simulink model "Pedal_Interpretation_exe"  (Simulink 7.0)
settings: Solver=ode4  StartTime=0.0  StopTime=88  FixedStep=0.01  RelTol=1e-3
InitFcn:
  | PedalInterp_para
values from neighbouring files (symbols this model uses):
  ped_min = 5    [PedalInterp_para.m]
  T_max_Brake = 4000    [PedalInterp_para.m]
  TI = 0    [PAS_callback.m]
undefined symbols (not defined in the file or in its folder): fzgbib, m_ab_100pro, m_ab_70pro, PedalInterpretation, v_bereich
libraries: simulink x320
(part 4 of 23)

== system Pedal_Interpretation_exe/TestData 1/SR-PI-02.2 Acceleration pedal interpretation/v = const & phi_Acc = const/Generate constant 6 ==
  Generate  constant for partition1 variant1 1 : Subsystem  mask(Feature generation){X0=0, T=2}
      mask prompts: X0 "Constant value:"; T "Duration"
      mask help: Output a decreasing ramp signal limited from bottom and top, starting at the specified time.
      mask Display: plot([1:2],[4,4])
  Generate  constant for partition1 variant2 1 : Subsystem  mask(Feature generation){X0=100, T=2}
      mask prompts: X0 "Constant value:"; T "Duration"
      mask help: Output a decreasing ramp signal limited from bottom and top, starting at the specified time.
      mask Display: plot([1:2],[4,4])
  Generate  constant for partition1 variant3 1 : Subsystem  mask(Feature generation){X0=50, T=2}
      mask prompts: X0 "Constant value:"; T "Duration"
      mask help: Output a decreasing ramp signal limited from bottom and top, starting at the specified time.
      mask Display: plot([1:2],[4,4])
  TestDataVariants Sequence : Subsystem
  switch : MultiPortSwitch  Inputs=3  OutDataType=sfix(16)  OutScaling=2^0
  phi_Acc : Outport  OutDataType=sfix(16)  OutScaling=2^0
  wires:
  switch/1 -> phi_Acc/1
  Generate  constant for partition1 variant2 1/1(Out1) -> switch/3
  Generate  constant for partition1 variant1 1/1(Out1) -> switch/2
  Generate  constant for partition1 variant3 1/1(Out1) -> switch/4
  TestDataVariants Sequence/1(Out1) -> switch/1

== system Pedal_Interpretation_exe/TestData 1/SR-PI-02.2 Acceleration pedal interpretation/v = const & phi_Acc decreases & T_des_Drive < 0/Bound Precond2 ==
  Signal : Inport  OutDataType=sfix(16)  OutScaling=2^0
  Reference : Inport  Port=2  OutDataType=sfix(16)  OutScaling=2^0
  RelOp : RelationalOperator  Operator=<  LogicOutDataTypeMode=Specify via dialog
  Activate : Outport  OutDataType=sfix(16)  OutScaling=2^0
  wires:
  Signal/1 -> RelOp/1
  RelOp/1 -> Activate/1
  Reference/1 -> RelOp/2

== system Pedal_Interpretation_exe/TestData 1/SR-PI-02.2 Acceleration pedal interpretation/v = const & phi_Acc decreases & T_des_Drive < 0/Generate constant 6 ==
  Generate  constant for partition1 variant1 1 : Subsystem  mask(Feature generation){X0=-10, T=2}
      mask prompts: X0 "Constant value:"; T "Duration"
      mask help: Output a decreasing ramp signal limited from bottom and top, starting at the specified time.
      mask Display: plot([1:2],[4,4])
  Generate  constant for partition1 variant2 1 : Subsystem  mask(Feature generation){X0=70, T=2}
      mask prompts: X0 "Constant value:"; T "Duration"
      mask help: Output a decreasing ramp signal limited from bottom and top, starting at the specified time.
      mask Display: plot([1:2],[4,4])
  Generate  constant for partition1 variant3 1 : Subsystem  mask(Feature generation){X0=0, T=2}
      mask prompts: X0 "Constant value:"; T "Duration"
      mask help: Output a decreasing ramp signal limited from bottom and top, starting at the specified time.
      mask Display: plot([1:2],[4,4])
  Generate  constant for partition1 variant4 1 : Subsystem  mask(Feature generation){X0=-5, T=2}
      mask prompts: X0 "Constant value:"; T "Duration"
      mask help: Output a decreasing ramp signal limited from bottom and top, starting at the specified time.
      mask Display: plot([1:2],[4,4])
  Generate  constant for partition1 variant5 1 : Subsystem  mask(Feature generation){X0=35, T=2}
      mask prompts: X0 "Constant value:"; T "Duration"
      mask help: Output a decreasing ramp signal limited from bottom and top, starting at the specified time.
      mask Display: plot([1:2],[4,4])
  TestDataVariants Sequence : Subsystem
  switch : MultiPortSwitch  Inputs=5  OutDataType=sfix(16)  OutScaling=2^0
  v_Fzg : Outport  OutDataType=sfix(16)  OutScaling=2^0
  wires:
  switch/1 -> v_Fzg/1
  Generate  constant for partition1 variant2 1/1(Out1) -> switch/3
  Generate  constant for partition1 variant1 1/1(Out1) -> switch/2
  Generate  constant for partition1 variant3 1/1(Out1) -> switch/4
  Generate  constant for partition1 variant4 1/1(Out1) -> switch/5
  Generate  constant for partition1 variant5 1/1(Out1) -> switch/6
  TestDataVariants Sequence/1(Out1) -> switch/1

== system Pedal_Interpretation_exe/TestData 1/SR-PI-02.2 Acceleration pedal interpretation/v = const & phi_Acc decreases & T_des_Drive < 0/Generate decrease 7 ==
  Generate  limited decrease for partition1 variant1 1 : Subsystem  mask(Feature generation){X0=10, XF=0, T=2}
      mask prompts: X0 "Initial output:"; XF "Final output:"; T "Duration"
      mask help: Output a decreasing ramp signal limited from bottom and top, starting at the specified time.
      mask Display:
      | plot([1:10],[4,4,4,4,4,1,1,1,1,1])
      | plot([1:10],[4,4,4,1,1,1,1,1,1,1])
      | plot([1:10],[4,1,1,1,1,1,1,1,1,1])
      | plot([1:10],[4,4,4,4,4,1,1,1,1,1])
      | plot([1:10],[4,4,4,4,4,4,4,1,1,1])
      | plot([1:10],[4,4,4,4,4,4,4,4,4,1])
      | plot([1:10],[4,4,4,4,4,4,4,4,4,4])
      | color('white');
      | plot([1:10],[1,1,1,1,1,1,1,1,1,1])
      | color('black');
      | plot([1,1.5],[1,1])
      | plot([2.5,3.5],[1,1])
      | plot([4.5,5.5],[1,1])
      | plot([6.5,7.5],[1,1])
      | plot([8.5,9.5],[1,1])
      | color('white');
      | plot([1,1.5],[4,4])
      | plot([2.5,3.5],[4,4])
      | plot([4.5,5.5],[4,4])
      | plot([6.5,7.5],[4,4])
      | plot([8.5,9.5],[4,4])
  Generate  limited decrease for partition1 variant2 1 : Subsystem  mask(Feature generation){X0=100, XF=90, T=2}
      mask prompts: X0 "Initial output:"; XF "Final output:"; T "Duration"
      mask help: Output a decreasing ramp signal limited from bottom and top, starting at the specified time.
      mask Display:
      | plot([1:10],[4,4,4,4,4,1,1,1,1,1])
      | plot([1:10],[4,4,4,1,1,1,1,1,1,1])
      | plot([1:10],[4,1,1,1,1,1,1,1,1,1])
      | plot([1:10],[4,4,4,4,4,1,1,1,1,1])
      | plot([1:10],[4,4,4,4,4,4,4,1,1,1])
      | plot([1:10],[4,4,4,4,4,4,4,4,4,1])
      | plot([1:10],[4,4,4,4,4,4,4,4,4,4])
      | color('white');
      | plot([1:10],[1,1,1,1,1,1,1,1,1,1])
      | color('black');
      | plot([1,1.5],[1,1])
      | plot([2.5,3.5],[1,1])
      | plot([4.5,5.5],[1,1])
      | plot([6.5,7.5],[1,1])
      | plot([8.5,9.5],[1,1])
      | color('white');
      | plot([1,1.5],[4,4])
      | plot([2.5,3.5],[4,4])
      | plot([4.5,5.5],[4,4])
      | plot([6.5,7.5],[4,4])
      | plot([8.5,9.5],[4,4])
  TestDataVariants Sequence : Subsystem
  switch : MultiPortSwitch  Inputs=2  OutDataType=sfix(16)  OutScaling=2^0
  phi_Acc : Outport  OutDataType=sfix(16)  OutScaling=2^0
  wires:
  switch/1 -> phi_Acc/1
  Generate  limited decrease for partition1 variant2 1/1(Out1) -> switch/3
  Generate  limited decrease for partition1 variant1 1/1(Out1) -> switch/2
  TestDataVariants Sequence/1(Out1) -> switch/1

== system Pedal_Interpretation_exe/TestData 1/SR-PI-02.2 Acceleration pedal interpretation/v = const & phi_Acc decreases & T_des_Drive >= 0/Bound Precond2 ==
  Signal : Inport  OutDataType=sfix(16)  OutScaling=2^0
  Reference : Inport  Port=2  OutDataType=sfix(16)  OutScaling=2^0
  RelOp : RelationalOperator  LogicOutDataTypeMode=Specify via dialog
  Activate : Outport  OutDataType=sfix(16)  OutScaling=2^0
  wires:
  Signal/1 -> RelOp/1
  RelOp/1 -> Activate/1
  Reference/1 -> RelOp/2

== system Pedal_Interpretation_exe/TestData 1/SR-PI-02.2 Acceleration pedal interpretation/v = const & phi_Acc decreases & T_des_Drive >= 0/Generate constant 6 ==
  Generate  constant for partition1 variant1 1 : Subsystem  mask(Feature generation){X0=-10, T=2}
      mask prompts: X0 "Constant value:"; T "Duration"
      mask help: Output a decreasing ramp signal limited from bottom and top, starting at the specified time.
      mask Display: plot([1:2],[4,4])
  Generate  constant for partition1 variant2 1 : Subsystem  mask(Feature generation){X0=70, T=2}
      mask prompts: X0 "Constant value:"; T "Duration"
      mask help: Output a decreasing ramp signal limited from bottom and top, starting at the specified time.
      mask Display: plot([1:2],[4,4])
  Generate  constant for partition1 variant3 1 : Subsystem  mask(Feature generation){X0=0, T=2}
      mask prompts: X0 "Constant value:"; T "Duration"
      mask help: Output a decreasing ramp signal limited from bottom and top, starting at the specified time.
      mask Display: plot([1:2],[4,4])
  Generate  constant for partition1 variant4 1 : Subsystem  mask(Feature generation){X0=-5, T=2}
      mask prompts: X0 "Constant value:"; T "Duration"
      mask help: Output a decreasing ramp signal limited from bottom and top, starting at the specified time.
      mask Display: plot([1:2],[4,4])
  Generate  constant for partition1 variant5 1 : Subsystem  mask(Feature generation){X0=35, T=2}
      mask prompts: X0 "Constant value:"; T "Duration"
      mask help: Output a decreasing ramp signal limited from bottom and top, starting at the specified time.
      mask Display: plot([1:2],[4,4])
  TestDataVariants Sequence : Subsystem
  switch : MultiPortSwitch  Inputs=5  OutDataType=sfix(16)  OutScaling=2^0
  v_Fzg : Outport  OutDataType=sfix(16)  OutScaling=2^0
  wires:
  switch/1 -> v_Fzg/1
  Generate  constant for partition1 variant2 1/1(Out1) -> switch/3
  Generate  constant for partition1 variant1 1/1(Out1) -> switch/2
  Generate  constant for partition1 variant3 1/1(Out1) -> switch/4
  Generate  constant for partition1 variant4 1/1(Out1) -> switch/5
  Generate  constant for partition1 variant5 1/1(Out1) -> switch/6
  TestDataVariants Sequence/1(Out1) -> switch/1

== system Pedal_Interpretation_exe/TestData 1/SR-PI-02.2 Acceleration pedal interpretation/v = const & phi_Acc decreases & T_des_Drive >= 0/Generate decrease 7 ==
  Generate  limited decrease for partition1 variant1 1 : Subsystem  mask(Feature generation){X0=10, XF=0, T=2}
      mask prompts: X0 "Initial output:"; XF "Final output:"; T "Duration"
      mask help: Output a decreasing ramp signal limited from bottom and top, starting at the specified time.
      mask Display:
      | plot([1:10],[4,4,4,4,4,1,1,1,1,1])
      | plot([1:10],[4,4,4,1,1,1,1,1,1,1])
      | plot([1:10],[4,1,1,1,1,1,1,1,1,1])
      | plot([1:10],[4,4,4,4,4,1,1,1,1,1])
      | plot([1:10],[4,4,4,4,4,4,4,1,1,1])
      | plot([1:10],[4,4,4,4,4,4,4,4,4,1])
      | plot([1:10],[4,4,4,4,4,4,4,4,4,4])
      | color('white');
      | plot([1:10],[1,1,1,1,1,1,1,1,1,1])
      | color('black');
      | plot([1,1.5],[1,1])
      | plot([2.5,3.5],[1,1])
      | plot([4.5,5.5],[1,1])
      | plot([6.5,7.5],[1,1])
      | plot([8.5,9.5],[1,1])
      | color('white');
      | plot([1,1.5],[4,4])
      | plot([2.5,3.5],[4,4])
      | plot([4.5,5.5],[4,4])
      | plot([6.5,7.5],[4,4])
      | plot([8.5,9.5],[4,4])
  Generate  limited decrease for partition1 variant2 1 : Subsystem  mask(Feature generation){X0=100, XF=90, T=2}
      mask prompts: X0 "Initial output:"; XF "Final output:"; T "Duration"
      mask help: Output a decreasing ramp signal limited from bottom and top, starting at the specified time.
      mask Display:
      | plot([1:10],[4,4,4,4,4,1,1,1,1,1])
      | plot([1:10],[4,4,4,1,1,1,1,1,1,1])
      | plot([1:10],[4,1,1,1,1,1,1,1,1,1])
      | plot([1:10],[4,4,4,4,4,1,1,1,1,1])
      | plot([1:10],[4,4,4,4,4,4,4,1,1,1])
      | plot([1:10],[4,4,4,4,4,4,4,4,4,1])
      | plot([1:10],[4,4,4,4,4,4,4,4,4,4])
      | color('white');
      | plot([1:10],[1,1,1,1,1,1,1,1,1,1])
      | color('black');
      | plot([1,1.5],[1,1])
      | plot([2.5,3.5],[1,1])
      | plot([4.5,5.5],[1,1])
      | plot([6.5,7.5],[1,1])
      | plot([8.5,9.5],[1,1])
      | color('white');
      | plot([1,1.5],[4,4])
      | plot([2.5,3.5],[4,4])
      | plot([4.5,5.5],[4,4])
      | plot([6.5,7.5],[4,4])
      | plot([8.5,9.5],[4,4])
  TestDataVariants Sequence : Subsystem
  switch : MultiPortSwitch  Inputs=2  OutDataType=sfix(16)  OutScaling=2^0
  phi_Acc : Outport  OutDataType=sfix(16)  OutScaling=2^0
  wires:
  switch/1 -> phi_Acc/1
  Generate  limited decrease for partition1 variant2 1/1(Out1) -> switch/3
  Generate  limited decrease for partition1 variant1 1/1(Out1) -> switch/2
  TestDataVariants Sequence/1(Out1) -> switch/1

== system Pedal_Interpretation_exe/TestData 1/SR-PI-02.2 Acceleration pedal interpretation/v = const & phi_Acc increases & T_des_Drive < 0/Bound Precond2 ==
  Signal : Inport  OutDataType=sfix(16)  OutScaling=2^0
  Reference : Inport  Port=2  OutDataType=sfix(16)  OutScaling=2^0
  RelOp : RelationalOperator  Operator=<  LogicOutDataTypeMode=Specify via dialog
  Activate : Outport  OutDataType=sfix(16)  OutScaling=2^0
  wires:
  Signal/1 -> RelOp/1
  RelOp/1 -> Activate/1
  Reference/1 -> RelOp/2

== system Pedal_Interpretation_exe/TestData 1/SR-PI-02.2 Acceleration pedal interpretation/v = const & phi_Acc increases & T_des_Drive < 0/Generate constant 6 ==
  Generate  constant for partition1 variant1 1 : Subsystem  mask(Feature generation){X0=-10, T=2}
      mask prompts: X0 "Constant value:"; T "Duration"
      mask help: Output a decreasing ramp signal limited from bottom and top, starting at the specified time.
      mask Display: plot([1:2],[4,4])
  Generate  constant for partition1 variant2 1 : Subsystem  mask(Feature generation){X0=70, T=2}
      mask prompts: X0 "Constant value:"; T "Duration"
      mask help: Output a decreasing ramp signal limited from bottom and top, starting at the specified time.
      mask Display: plot([1:2],[4,4])
  Generate  constant for partition1 variant3 1 : Subsystem  mask(Feature generation){X0=0, T=2}
      mask prompts: X0 "Constant value:"; T "Duration"
      mask help: Output a decreasing ramp signal limited from bottom and top, starting at the specified time.
      mask Display: plot([1:2],[4,4])
  Generate  constant for partition1 variant4 1 : Subsystem  mask(Feature generation){X0=-5, T=2}
      mask prompts: X0 "Constant value:"; T "Duration"
      mask help: Output a decreasing ramp signal limited from bottom and top, starting at the specified time.
      mask Display: plot([1:2],[4,4])
  Generate  constant for partition1 variant5 1 : Subsystem  mask(Feature generation){X0=35, T=2}
      mask prompts: X0 "Constant value:"; T "Duration"
      mask help: Output a decreasing ramp signal limited from bottom and top, starting at the specified time.
      mask Display: plot([1:2],[4,4])
  TestDataVariants Sequence : Subsystem
  switch : MultiPortSwitch  Inputs=5  OutDataType=sfix(16)  OutScaling=2^0
  v_Fzg : Outport  OutDataType=sfix(16)  OutScaling=2^0
  wires:
  switch/1 -> v_Fzg/1
  Generate  constant for partition1 variant2 1/1(Out1) -> switch/3
  Generate  constant for partition1 variant1 1/1(Out1) -> switch/2
  Generate  constant for partition1 variant3 1/1(Out1) -> switch/4
  Generate  constant for partition1 variant4 1/1(Out1) -> switch/5
  Generate  constant for partition1 variant5 1/1(Out1) -> switch/6
  TestDataVariants Sequence/1(Out1) -> switch/1

== system Pedal_Interpretation_exe/TestData 1/SR-PI-02.2 Acceleration pedal interpretation/v = const & phi_Acc increases & T_des_Drive < 0/Generate increase 7 ==
  Generate  limited increase for partition1 variant1 1 : Subsystem  mask(Feature generation){X0=0, XF=10, T=2}
      mask prompts: X0 "Initial output:"; XF "Final output:"; T "Duration:"
      mask help: Output a ramp signal limited from bottom and top, starting at the specified time.
      mask Display:
      | plot([1:10],[1,1,1,1,1,4,4,4,4,4])
      | plot([1:10],[1,4,4,4,4,4,4,4,4,4])
      | plot([1:10],[1,1,1,4,4,4,4,4,4,4])
      | plot([1:10],[1,1,1,1,1,4,4,4,4,4])
      | plot([1:10],[1,1,1,1,1,1,1,4,4,4])
      | plot([1:10],[1,1,1,1,1,1,1,1,1,4])
      | plot([5:10],[1,1,1,1,1,1])
      | color('white');
      | plot([1:10],[4,4,4,4,4,4,4,4,4,4])
      | color('white');
      | plot([1,1.5],[1,1])
      | plot([2.5,3.5],[1,1])
      | plot([4.5,5.5],[1,1])
      | plot([6.5,7.5],[1,1])
      | plot([8.5,9.5],[1,1])
      | color('black');
      | plot([1,1.5],[4,4])
      | plot([2.5,3.5],[4,4])
      | plot([4.5,5.5],[4,4])
      | plot([6.5,7.5],[4,4])
      | plot([8.5,9.5],[4,4])
  Generate  limited increase for partition1 variant2 1 : Subsystem  mask(Feature generation){X0=90, XF=100, T=2}
      mask prompts: X0 "Initial output:"; XF "Final output:"; T "Duration:"
      mask help: Output a ramp signal limited from bottom and top, starting at the specified time.
      mask Display:
      | plot([1:10],[1,1,1,1,1,4,4,4,4,4])
      | plot([1:10],[1,4,4,4,4,4,4,4,4,4])
      | plot([1:10],[1,1,1,4,4,4,4,4,4,4])
      | plot([1:10],[1,1,1,1,1,4,4,4,4,4])
      | plot([1:10],[1,1,1,1,1,1,1,4,4,4])
      | plot([1:10],[1,1,1,1,1,1,1,1,1,4])
      | plot([5:10],[1,1,1,1,1,1])
      | color('white');
      | plot([1:10],[4,4,4,4,4,4,4,4,4,4])
      | color('white');
      | plot([1,1.5],[1,1])
      | plot([2.5,3.5],[1,1])
      | plot([4.5,5.5],[1,1])
      | plot([6.5,7.5],[1,1])
      | plot([8.5,9.5],[1,1])
      | color('black');
      | plot([1,1.5],[4,4])
      | plot([2.5,3.5],[4,4])
      | plot([4.5,5.5],[4,4])
      | plot([6.5,7.5],[4,4])
      | plot([8.5,9.5],[4,4])
  TestDataVariants Sequence : Subsystem
  switch : MultiPortSwitch  Inputs=2  OutDataType=sfix(16)  OutScaling=2^0
  phi_Acc : Outport  OutDataType=sfix(16)  OutScaling=2^0
  wires:
  switch/1 -> phi_Acc/1
  Generate  limited increase for partition1 variant2 1/1(Out1) -> switch/3
  Generate  limited increase for partition1 variant1 1/1(Out1) -> switch/2
  TestDataVariants Sequence/1(Out1) -> switch/1

== system Pedal_Interpretation_exe/TestData 1/SR-PI-02.2 Acceleration pedal interpretation/v = const & phi_Acc increases & T_des_Drive >= 0/Bound Precond2 ==
  Signal : Inport  OutDataType=sfix(16)  OutScaling=2^0
  Reference : Inport  Port=2  OutDataType=sfix(16)  OutScaling=2^0
  RelOp : RelationalOperator  LogicOutDataTypeMode=Specify via dialog
  Activate : Outport  OutDataType=sfix(16)  OutScaling=2^0
  wires:
  Signal/1 -> RelOp/1
  RelOp/1 -> Activate/1
  Reference/1 -> RelOp/2

== system Pedal_Interpretation_exe/TestData 1/SR-PI-02.2 Acceleration pedal interpretation/v = const & phi_Acc increases & T_des_Drive >= 0/Generate constant 6 ==
  Generate  constant for partition1 variant1 1 : Subsystem  mask(Feature generation){X0=-10, T=2}
      mask prompts: X0 "Constant value:"; T "Duration"
      mask help: Output a decreasing ramp signal limited from bottom and top, starting at the specified time.
      mask Display: plot([1:2],[4,4])
  Generate  constant for partition1 variant2 1 : Subsystem  mask(Feature generation){X0=70, T=2}
      mask prompts: X0 "Constant value:"; T "Duration"
      mask help: Output a decreasing ramp signal limited from bottom and top, starting at the specified time.
      mask Display: plot([1:2],[4,4])
  Generate  constant for partition1 variant3 1 : Subsystem  mask(Feature generation){X0=0, T=2}
      mask prompts: X0 "Constant value:"; T "Duration"
      mask help: Output a decreasing ramp signal limited from bottom and top, starting at the specified time.
      mask Display: plot([1:2],[4,4])
  Generate  constant for partition1 variant4 1 : Subsystem  mask(Feature generation){X0=-5, T=2}
      mask prompts: X0 "Constant value:"; T "Duration"
      mask help: Output a decreasing ramp signal limited from bottom and top, starting at the specified time.
      mask Display: plot([1:2],[4,4])
  Generate  constant for partition1 variant5 1 : Subsystem  mask(Feature generation){X0=35, T=2}
      mask prompts: X0 "Constant value:"; T "Duration"
      mask help: Output a decreasing ramp signal limited from bottom and top, starting at the specified time.
      mask Display: plot([1:2],[4,4])
  TestDataVariants Sequence : Subsystem
  switch : MultiPortSwitch  Inputs=5  OutDataType=sfix(16)  OutScaling=2^0
  v_Fzg : Outport  OutDataType=sfix(16)  OutScaling=2^0
  wires:
  switch/1 -> v_Fzg/1
  Generate  constant for partition1 variant2 1/1(Out1) -> switch/3
  Generate  constant for partition1 variant1 1/1(Out1) -> switch/2
  Generate  constant for partition1 variant3 1/1(Out1) -> switch/4
  Generate  constant for partition1 variant4 1/1(Out1) -> switch/5
  Generate  constant for partition1 variant5 1/1(Out1) -> switch/6
  TestDataVariants Sequence/1(Out1) -> switch/1

== system Pedal_Interpretation_exe/TestData 1/SR-PI-02.2 Acceleration pedal interpretation/v = const & phi_Acc increases & T_des_Drive >= 0/Generate increase 7 ==
  Generate  limited increase for partition1 variant1 1 : Subsystem  mask(Feature generation){X0=0, XF=10, T=2}
      mask prompts: X0 "Initial output:"; XF "Final output:"; T "Duration:"
      mask help: Output a ramp signal limited from bottom and top, starting at the specified time.
      mask Display:
      | plot([1:10],[1,1,1,1,1,4,4,4,4,4])
      | plot([1:10],[1,4,4,4,4,4,4,4,4,4])
      | plot([1:10],[1,1,1,4,4,4,4,4,4,4])
      | plot([1:10],[1,1,1,1,1,4,4,4,4,4])
      | plot([1:10],[1,1,1,1,1,1,1,4,4,4])
      | plot([1:10],[1,1,1,1,1,1,1,1,1,4])
      | plot([5:10],[1,1,1,1,1,1])
      | color('white');
      | plot([1:10],[4,4,4,4,4,4,4,4,4,4])
      | color('white');
      | plot([1,1.5],[1,1])
      | plot([2.5,3.5],[1,1])
      | plot([4.5,5.5],[1,1])
      | plot([6.5,7.5],[1,1])
      | plot([8.5,9.5],[1,1])
      | color('black');
      | plot([1,1.5],[4,4])
      | plot([2.5,3.5],[4,4])
      | plot([4.5,5.5],[4,4])
      | plot([6.5,7.5],[4,4])
      | plot([8.5,9.5],[4,4])
  Generate  limited increase for partition1 variant2 1 : Subsystem  mask(Feature generation){X0=90, XF=100, T=2}
      mask prompts: X0 "Initial output:"; XF "Final output:"; T "Duration:"
      mask help: Output a ramp signal limited from bottom and top, starting at the specified time.
      mask Display:
      | plot([1:10],[1,1,1,1,1,4,4,4,4,4])
      | plot([1:10],[1,4,4,4,4,4,4,4,4,4])
      | plot([1:10],[1,1,1,4,4,4,4,4,4,4])
      | plot([1:10],[1,1,1,1,1,4,4,4,4,4])
      | plot([1:10],[1,1,1,1,1,1,1,4,4,4])
      | plot([1:10],[1,1,1,1,1,1,1,1,1,4])
      | plot([5:10],[1,1,1,1,1,1])
      | color('white');
      | plot([1:10],[4,4,4,4,4,4,4,4,4,4])
      | color('white');
      | plot([1,1.5],[1,1])
      | plot([2.5,3.5],[1,1])
      | plot([4.5,5.5],[1,1])
      | plot([6.5,7.5],[1,1])
      | plot([8.5,9.5],[1,1])
      | color('black');
      | plot([1,1.5],[4,4])
      | plot([2.5,3.5],[4,4])
      | plot([4.5,5.5],[4,4])
      | plot([6.5,7.5],[4,4])
      | plot([8.5,9.5],[4,4])
  TestDataVariants Sequence : Subsystem
  switch : MultiPortSwitch  Inputs=2  OutDataType=sfix(16)  OutScaling=2^0
  phi_Acc : Outport  OutDataType=sfix(16)  OutScaling=2^0
  wires:
  switch/1 -> phi_Acc/1
  Generate  limited increase for partition1 variant2 1/1(Out1) -> switch/3
  Generate  limited increase for partition1 variant1 1/1(Out1) -> switch/2
  TestDataVariants Sequence/1(Out1) -> switch/1

== system Pedal_Interpretation_exe/TestData 1/SR-PI-02.2 Acceleration pedal interpretation/v increases & phi_Acc = const & T_des_Drive >= 0/Bound Precond2 ==
  Signal : Inport  OutDataType=sfix(16)  OutScaling=2^0
  Reference : Inport  Port=2  OutDataType=sfix(16)  OutScaling=2^0
  RelOp : RelationalOperator  LogicOutDataTypeMode=Specify via dialog
  Activate : Outport  OutDataType=sfix(16)  OutScaling=2^0
  wires:
  Signal/1 -> RelOp/1
  RelOp/1 -> Activate/1
  Reference/1 -> RelOp/2

== system Pedal_Interpretation_exe/TestData 1/SR-PI-02.2 Acceleration pedal interpretation/v increases & phi_Acc = const & T_des_Drive >= 0/Generate constant 6 ==
  Generate  constant for partition1 variant1 1 : Subsystem  mask(Feature generation){X0=0, T=2}
      mask prompts: X0 "Constant value:"; T "Duration"
      mask help: Output a decreasing ramp signal limited from bottom and top, starting at the specified time.
      mask Display: plot([1:2],[4,4])
  Generate  constant for partition1 variant2 1 : Subsystem  mask(Feature generation){X0=100, T=2}
      mask prompts: X0 "Constant value:"; T "Duration"
      mask help: Output a decreasing ramp signal limited from bottom and top, starting at the specified time.
      mask Display: plot([1:2],[4,4])
  Generate  constant for partition1 variant3 1 : Subsystem  mask(Feature generation){X0=50, T=2}
      mask prompts: X0 "Constant value:"; T "Duration"
      mask help: Output a decreasing ramp signal limited from bottom and top, starting at the specified time.
      mask Display: plot([1:2],[4,4])
  TestDataVariants Sequence : Subsystem
  switch : MultiPortSwitch  Inputs=3  OutDataType=sfix(16)  OutScaling=2^0
  phi_Acc : Outport  OutDataType=sfix(16)  OutScaling=2^0
  wires:
  switch/1 -> phi_Acc/1
  Generate  constant for partition1 variant2 1/1(Out1) -> switch/3
  Generate  constant for partition1 variant1 1/1(Out1) -> switch/2
  Generate  constant for partition1 variant3 1/1(Out1) -> switch/4
  TestDataVariants Sequence/1(Out1) -> switch/1

== system Pedal_Interpretation_exe/TestData 1/SR-PI-02.2 Acceleration pedal interpretation/v increases & phi_Acc = const & T_des_Drive >= 0/Generate increase 7 ==
  Generate  limited increase for partition1 variant1 1 : Subsystem  mask(Feature generation){X0=-10, XF=-9, T=2}
      mask prompts: X0 "Initial output:"; XF "Final output:"; T "Duration:"
      mask help: Output a ramp signal limited from bottom and top, starting at the specified time.
      mask Display:
      | plot([1:10],[1,1,1,1,1,4,4,4,4,4])
      | plot([1:10],[1,4,4,4,4,4,4,4,4,4])
      | plot([1:10],[1,1,1,4,4,4,4,4,4,4])
      | plot([1:10],[1,1,1,1,1,4,4,4,4,4])
      | plot([1:10],[1,1,1,1,1,1,1,4,4,4])
      | plot([1:10],[1,1,1,1,1,1,1,1,1,4])
      | plot([5:10],[1,1,1,1,1,1])
      | color('white');
      | plot([1:10],[4,4,4,4,4,4,4,4,4,4])
      | color('white');
      | plot([1,1.5],[1,1])
      | plot([2.5,3.5],[1,1])
      | plot([4.5,5.5],[1,1])
      | plot([6.5,7.5],[1,1])
      | plot([8.5,9.5],[1,1])
      | color('black');
      | plot([1,1.5],[4,4])
      | plot([2.5,3.5],[4,4])
      | plot([4.5,5.5],[4,4])
      | plot([6.5,7.5],[4,4])
      | plot([8.5,9.5],[4,4])
  Generate  limited increase for partition1 variant2 1 : Subsystem  mask(Feature generation){X0=-1, XF=0, T=2}
      mask prompts: X0 "Initial output:"; XF "Final output:"; T "Duration:"
      mask help: Output a ramp signal limited from bottom and top, starting at the specified time.
      mask Display:
      | plot([1:10],[1,1,1,1,1,4,4,4,4,4])
      | plot([1:10],[1,4,4,4,4,4,4,4,4,4])
      | plot([1:10],[1,1,1,4,4,4,4,4,4,4])
      | plot([1:10],[1,1,1,1,1,4,4,4,4,4])
      | plot([1:10],[1,1,1,1,1,1,1,4,4,4])
      | plot([1:10],[1,1,1,1,1,1,1,1,1,4])
      | plot([5:10],[1,1,1,1,1,1])
      | color('white');
      | plot([1:10],[4,4,4,4,4,4,4,4,4,4])
      | color('white');
      | plot([1,1.5],[1,1])
      | plot([2.5,3.5],[1,1])
      | plot([4.5,5.5],[1,1])
      | plot([6.5,7.5],[1,1])
      | plot([8.5,9.5],[1,1])
      | color('black');
      | plot([1,1.5],[4,4])
      | plot([2.5,3.5],[4,4])
      | plot([4.5,5.5],[4,4])
      | plot([6.5,7.5],[4,4])
      | plot([8.5,9.5],[4,4])
  Generate  limited increase for partition2 variant1 1 : Subsystem  mask(Feature generation){X0=0, XF=7, T=2}
      mask prompts: X0 "Initial output:"; XF "Final output:"; T "Duration:"
      mask help: Output a ramp signal limited from bottom and top, starting at the specified time.
      mask Display:
      | plot([1:10],[1,1,1,1,1,4,4,4,4,4])
      | plot([1:10],[1,4,4,4,4,4,4,4,4,4])
      | plot([1:10],[1,1,1,4,4,4,4,4,4,4])
      | plot([1:10],[1,1,1,1,1,4,4,4,4,4])
      | plot([1:10],[1,1,1,1,1,1,1,4,4,4])
      | plot([1:10],[1,1,1,1,1,1,1,1,1,4])
      | plot([5:10],[1,1,1,1,1,1])
      | color('white');
      | plot([1:10],[4,4,4,4,4,4,4,4,4,4])
      | color('white');
      | plot([1,1.5],[1,1])
      | plot([2.5,3.5],[1,1])
      | plot([4.5,5.5],[1,1])
      | plot([6.5,7.5],[1,1])
      | plot([8.5,9.5],[1,1])
      | color('black');
      | plot([1,1.5],[4,4])
      | plot([2.5,3.5],[4,4])
      | plot([4.5,5.5],[4,4])
      | plot([6.5,7.5],[4,4])
      | plot([8.5,9.5],[4,4])
  Generate  limited increase for partition2 variant2 1 : Subsystem  mask(Feature generation){X0=63, XF=70, T=2}
      mask prompts: X0 "Initial output:"; XF "Final output:"; T "Duration:"
      mask help: Output a ramp signal limited from bottom and top, starting at the specified time.
      mask Display:
      | plot([1:10],[1,1,1,1,1,4,4,4,4,4])
      | plot([1:10],[1,4,4,4,4,4,4,4,4,4])
      | plot([1:10],[1,1,1,4,4,4,4,4,4,4])
      | plot([1:10],[1,1,1,1,1,4,4,4,4,4])
      | plot([1:10],[1,1,1,1,1,1,1,4,4,4])
      | plot([1:10],[1,1,1,1,1,1,1,1,1,4])
      | plot([5:10],[1,1,1,1,1,1])
      | color('white');
      | plot([1:10],[4,4,4,4,4,4,4,4,4,4])
      | color('white');
      | plot([1,1.5],[1,1])
      | plot([2.5,3.5],[1,1])
      | plot([4.5,5.5],[1,1])
      | plot([6.5,7.5],[1,1])
      | plot([8.5,9.5],[1,1])
      | color('black');
      | plot([1,1.5],[4,4])
      | plot([2.5,3.5],[4,4])
      | plot([4.5,5.5],[4,4])
      | plot([6.5,7.5],[4,4])
      | plot([8.5,9.5],[4,4])
  TestDataVariants Sequence : Subsystem
  switch : MultiPortSwitch  OutDataType=sfix(16)  OutScaling=2^0
  v_Fzg : Outport  OutDataType=sfix(16)  OutScaling=2^0
  wires:
  switch/1 -> v_Fzg/1
  Generate  limited increase for partition1 variant2 1/1(Out1) -> switch/3
  Generate  limited increase for partition1 variant1 1/1(Out1) -> switch/2
  Generate  limited increase for partition2 variant2 1/1(Out1) -> switch/5
  Generate  limited increase for partition2 variant1 1/1(Out1) -> switch/4
  TestDataVariants Sequence/1(Out1) -> switch/1

== system Pedal_Interpretation_exe/Validation Functions/SR-PI-01.1 Brake Pedal recognition/BrakePedal == 0/PAS ==
  Precond : Inport  OutDataType=sfix(16)  OutScaling=2^0
  V : Inport  Port=2  OutDataType=sfix(16)  OutScaling=2^0
  A delay : Subsystem  TreatAsAtomicUnit=on  mask{Delay=0}
      mask prompts: Delay "Delay (in simulation steps) for the input signal:"
      mask init:
      | %set_param([gcb '/Discrete Transfer Fcn'],'Denominator',['[' num2str([1 zeros(1,str2double(get_param(gcb,'Delay')))]) ']']);
      mask CallbackString:
      | Delay = str2double(get_param(gcb,'Delay'));
      | if Delay < 0
      |     set_param(gcb,'Delay','0');
      |     error('Only non-negative delays are possible (causality).');
      |     set_param([gcb '/Delay'],'Value','0');
      | elseif Delay == 0
      |     set_param([gcb '/Delay'],'Value','0');
      | else
      |     set_param([gcb '/Integer Delay'],'NumDelays',num2str(Delay));
      |     set_param([gcb '/Delay'],'Value',num2str(Delay));
      | end
      mask Display: text(0.5,0.5,['z^{ ' num2str((-1)*str2double(get_param(gcb,'Delay'))) '}'],'texmode','on');
  AND1 : Logic  AllPortsSameDT=off  OutDataTypeMode=boolean
  Bus Selector : BusSelector  OutputSignals=Local verdict
  Bus Selector1 : BusSelector  OutputSignals=Expected lower limit,Expected upper limit,Actual data
  Bus Selector2 : BusSelector  OutputSignals=R,T,A
  Bus Assignment : BusAssignment  AssignedSignals=Local verdict,Delay
  Bus Assignment1 : BusAssignment  AssignedSignals=Expected lower limit,Expected upper limit,Actual data
  Constant : Constant  Value=-1  OutDataType=sfix(16)  OutScaling=2^0
  Delay bus signals : Subsystem
  Ra delay : Subsystem  TreatAsAtomicUnit=on  mask{Delay=0}
      mask prompts: Delay "Delay (in simulation steps) for the input signal:"
      mask init:
      | %set_param([gcb '/Discrete Transfer Fcn'],'Denominator',['[' num2str([1 zeros(1,str2double(get_param(gcb,'Delay')))]) ']']);
      mask CallbackString:
      | Delay = str2double(get_param(gcb,'Delay'));
      | if Delay < 0
      |     set_param(gcb,'Delay','0');
      |     error('Only non-negative delays are possible (causality).');
      |     set_param([gcb '/Delay'],'Value','0');
      | elseif Delay == 0
      |     set_param([gcb '/Delay'],'Value','0');
      | else
      |     set_param([gcb '/Integer Delay'],'NumDelays',num2str(Delay));
      |     set_param([gcb '/Delay'],'Value',num2str(Delay));
      | end
      mask Display: text(0.5,0.5,['z^{ ' num2str((-1)*str2double(get_param(gcb,'Delay'))) '}'],'texmode','on');
  Rp delay : Subsystem  TreatAsAtomicUnit=on  mask{Delay=0}
      mask prompts: Delay "Delay (in simulation steps) for the input signal:"
      mask init:
      | %set_param([gcb '/Discrete Transfer Fcn'],'Denominator',['[' num2str([1 zeros(1,str2double(get_param(gcb,'Delay')))]) ']']);
      mask CallbackString:
      | Delay = str2double(get_param(gcb,'Delay'));
      | if Delay < 0
      |     set_param(gcb,'Delay','0');
      |     error('Only non-negative delays are possible (causality).');
      |     set_param([gcb '/Delay'],'Value','0');
      | elseif Delay == 0
      |     set_param([gcb '/Delay'],'Value','0');
      | else
      |     set_param([gcb '/Integer Delay'],'NumDelays',num2str(Delay));
      |     set_param([gcb '/Delay'],'Value',num2str(Delay));
      | end
      mask Display: text(0.5,0.5,['z^{ ' num2str((-1)*str2double(get_param(gcb,'Delay'))) '}'],'texmode','on');
  Ta delay : Subsystem  TreatAsAtomicUnit=on  mask{Delay=0}
      mask prompts: Delay "Delay (in simulation steps) for the input signal:"
      mask init:
      | %set_param([gcb '/Discrete Transfer Fcn'],'Denominator',['[' num2str([1 zeros(1,str2double(get_param(gcb,'Delay')))]) ']']);
      mask CallbackString:
      | Delay = str2double(get_param(gcb,'Delay'));
      | if Delay < 0
      |     set_param(gcb,'Delay','0');
      |     error('Only non-negative delays are possible (causality).');
      |     set_param([gcb '/Delay'],'Value','0');
      | elseif Delay == 0
      |     set_param([gcb '/Delay'],'Value','0');
      | else
      |     set_param([gcb '/Integer Delay'],'NumDelays',num2str(Delay));
      |     set_param([gcb '/Delay'],'Value',num2str(Delay));
      | end
      mask Display: text(0.5,0.5,['z^{ ' num2str((-1)*str2double(get_param(gcb,'Delay'))) '}'],'texmode','on');
  Tp delay : Subsystem  TreatAsAtomicUnit=on  mask{Delay=0}
      mask prompts: Delay "Delay (in simulation steps) for the input signal:"
      mask init:
      | %set_param([gcb '/Discrete Transfer Fcn'],'Denominator',['[' num2str([1 zeros(1,str2double(get_param(gcb,'Delay')))]) ']']);
      mask CallbackString:
      | Delay = str2double(get_param(gcb,'Delay'));
      | if Delay < 0
      |     set_param(gcb,'Delay','0');
      |     error('Only non-negative delays are possible (causality).');
      |     set_param([gcb '/Delay'],'Value','0');
      | elseif Delay == 0
      |     set_param([gcb '/Delay'],'Value','0');
      | else
      |     set_param([gcb '/Integer Delay'],'NumDelays',num2str(Delay));
      |     set_param([gcb '/Delay'],'Value',num2str(Delay));
      | end
      mask Display: text(0.5,0.5,['z^{ ' num2str((-1)*str2double(get_param(gcb,'Delay'))) '}'],'texmode','on');
  V delay : Subsystem  TreatAsAtomicUnit=on  mask{Delay=0}
      mask prompts: Delay "Delay (in simulation steps) for the input signal:"
      mask init:
      | %set_param([gcb '/Discrete Transfer Fcn'],'Denominator',['[' num2str([1 zeros(1,str2double(get_param(gcb,'Delay')))]) ']']);
      mask CallbackString:
      | Delay = str2double(get_param(gcb,'Delay'));
      | if Delay < 0
      |     set_param(gcb,'Delay','0');
      |     error('Only non-negative delays are possible (causality).');
      |     set_param([gcb '/Delay'],'Value','0');
      | elseif Delay == 0
      |     set_param([gcb '/Delay'],'Value','0');
      | else
      |     set_param([gcb '/Integer Delay'],'NumDelays',num2str(Delay));
      |     set_param([gcb '/Delay'],'Value',num2str(Delay));
      | end
      mask Display: text(0.5,0.5,['z^{ ' num2str((-1)*str2double(get_param(gcb,'Delay'))) '}'],'texmode','on');
  error : Subsystem
  none - pass - fail : Subsystem
  sw D : Switch  Criteria=u2 ~= 0
  sw V : Switch  Criteria=u2 ~= 0
  VF Info : Outport  OutDataType=sfix(16)  OutScaling=2^0
  wires:
  V/1 -> Bus Selector/1, Bus Selector1/1, Bus Assignment1/1
  error/1(Verror) -> sw V/2, sw D/2
  Constant/1 -> sw V/1
  none - pass - fail/1(Verdict) -> sw V/3
  none - pass - fail/2(MaxDelay) -> sw D/1
  none - pass - fail/3(Delay) -> sw D/3
  sw V/1 -> Bus Assignment/2
  sw D/1 -> Bus Assignment/3
  Bus Selector/1 -> V delay/1(In1), Ra delay/1(In1), Ta delay/1(In1)  "<Local verdict>"
  Bus Assignment/1 -> VF Info/1
  Bus Selector2/1 -> Rp delay/1(In1)  "<R>"
  Bus Selector2/2 -> Tp delay/1(In1)  "<T>"
  Bus Selector2/3 -> A delay/1(In1)  "<A>"
  Rp delay/1(Out1) -> error/1(Rp), none - pass - fail/1(Rp), AND1/1
  Tp delay/1(Out1) -> error/2(Tp), none - pass - fail/2(Tp)
  A delay/1(Out1) -> error/3(A), none - pass - fail/3(A)
  V delay/1(Out1) -> error/6(V), none - pass - fail/6(V)
  Ra delay/1(Out1) -> none - pass - fail/4(Ra), AND1/2, error/4(Ra)
  AND1/1 -> none - pass - fail/7(R AND)
  Precond/1 -> Bus Selector2/1
  Bus Selector1/1 -> Delay bus signals/1(ELLin)  "<Expected lower limit>"
  Bus Selector1/2 -> Delay bus signals/2(EULin)  "<Expected upper limit>"
  Bus Selector1/3 -> Delay bus signals/3(ADin)  "<Actual data>"
  Bus Assignment1/1 -> Bus Assignment/1
  Delay bus signals/1(ELLout) -> Bus Assignment1/2
  Delay bus signals/2(EULout) -> Bus Assignment1/3
  Delay bus signals/3(ADout) -> Bus Assignment1/4
  Ta delay/1(Out1) -> none - pass - fail/5(Ta), error/5(Ta)

== system Pedal_Interpretation_exe/Validation Functions/SR-PI-01.1 Brake Pedal recognition/BrakePedal == 0/Range - Gap Relative tolerance Ass ==
  Signal : Inport  OutDataType=sfix(16)  OutScaling=2^0
  Reference : Inport  Port=2  OutDataType=sfix(16)  OutScaling=2^0
  Abs : Abs
  Abs1 : Abs
  Add : Sum  Inputs=+-  OutDataType=sfix(16)  OutScaling=2^-10
  Add1 : Sum  Inputs=+-  OutDataType=sfix(16)  OutScaling=2^-10
  Add2 : Sum  OutDataType=sfix(16)  OutScaling=2^-10
  Bus Creator : BusCreator  Inputs=5
  Data Type Conversion : DataTypeConversion  OutDataTypeMode=double  OutDataType=sfix(16)  OutScaling=2^0
  Data Type Conversion1 : DataTypeConversion  OutDataType=sfix(16)  OutScaling=2^0
  Data Type Conversion2 : DataTypeConversion  OutDataType=sfix(16)  OutScaling=2^0
  Data Type Conversion3 : DataTypeConversion  OutDataType=sfix(16)  OutScaling=2^0
  Delay : Constant  Value=0  OutDataType=sfix(16)  OutScaling=2^0
  Divide1 : Product  Inputs=**/  OutDataType=sfix(16)  OutScaling=2^-10
  Max : Constant  Value=100  OutDataType=sfix(16)  OutScaling=2^0
  Relational Operator : RelationalOperator  Operator=<=  LogicOutDataTypeMode=boolean
  Relative Tolerance : Constant  OutDataType=sfix(16)  OutScaling=2^0
  V : Outport  OutDataType=sfix(16)  OutScaling=2^0  InitialOutput=[2]
  wires:
  Data Type Conversion3/1 -> Bus Creator/4  "Actual data"
  Data Type Conversion2/1 -> Bus Creator/3  "Expected upper limit"
  Data Type Conversion1/1 -> Bus Creator/2  "Expected lower limit"
  Data Type Conversion/1 -> Bus Creator/1  "Local verdict"
  Bus Creator/1 -> V/1
  Add1/1 -> Data Type Conversion1/1
  Add2/1 -> Data Type Conversion2/1
  Delay/1 -> Bus Creator/5  "Delay"
  Abs1/1 -> Divide1/1
  Relational Operator/1 -> Data Type Conversion/1
  Relative Tolerance/1 -> Divide1/2
  Max/1 -> Divide1/3
  Divide1/1 -> Add2/1, Add1/2, Relational Operator/2
  Reference/1 -> Add1/1, Add2/2, Abs1/1, Add/2
  Signal/1 -> Data Type Conversion3/1, Add/1
  Add/1 -> Abs/1
  Abs/1 -> Relational Operator/1

== system Pedal_Interpretation_exe/Validation Functions/SR-PI-01.1 Brake Pedal recognition/BrakePedal == 1/PAS ==
  Precond : Inport  OutDataType=sfix(16)  OutScaling=2^0
  V : Inport  Port=2  OutDataType=sfix(16)  OutScaling=2^0
  A delay : Subsystem  TreatAsAtomicUnit=on  mask{Delay=0}
      mask prompts: Delay "Delay (in simulation steps) for the input signal:"
      mask init:
      | %set_param([gcb '/Discrete Transfer Fcn'],'Denominator',['[' num2str([1 zeros(1,str2double(get_param(gcb,'Delay')))]) ']']);
      mask CallbackString:
      | Delay = str2double(get_param(gcb,'Delay'));
      | if Delay < 0
      |     set_param(gcb,'Delay','0');
      |     error('Only non-negative delays are possible (causality).');
      |     set_param([gcb '/Delay'],'Value','0');
      | elseif Delay == 0
      |     set_param([gcb '/Delay'],'Value','0');
      | else
      |     set_param([gcb '/Integer Delay'],'NumDelays',num2str(Delay));
      |     set_param([gcb '/Delay'],'Value',num2str(Delay));
      | end
      mask Display: text(0.5,0.5,['z^{ ' num2str((-1)*str2double(get_param(gcb,'Delay'))) '}'],'texmode','on');
  AND1 : Logic  AllPortsSameDT=off  OutDataTypeMode=boolean
  Bus Selector : BusSelector  OutputSignals=Local verdict
  Bus Selector1 : BusSelector  OutputSignals=Expected lower limit,Expected upper limit,Actual data
  Bus Selector2 : BusSelector  OutputSignals=R,T,A
  Bus Assignment : BusAssignment  AssignedSignals=Local verdict,Delay
  Bus Assignment1 : BusAssignment  AssignedSignals=Expected lower limit,Expected upper limit,Actual data
  Constant : Constant  Value=-1  OutDataType=sfix(16)  OutScaling=2^0
  Delay bus signals : Subsystem
  Ra delay : Subsystem  TreatAsAtomicUnit=on  mask{Delay=0}
      mask prompts: Delay "Delay (in simulation steps) for the input signal:"
      mask init:
      | %set_param([gcb '/Discrete Transfer Fcn'],'Denominator',['[' num2str([1 zeros(1,str2double(get_param(gcb,'Delay')))]) ']']);
      mask CallbackString:
      | Delay = str2double(get_param(gcb,'Delay'));
      | if Delay < 0
      |     set_param(gcb,'Delay','0');
      |     error('Only non-negative delays are possible (causality).');
      |     set_param([gcb '/Delay'],'Value','0');
      | elseif Delay == 0
      |     set_param([gcb '/Delay'],'Value','0');
      | else
      |     set_param([gcb '/Integer Delay'],'NumDelays',num2str(Delay));
      |     set_param([gcb '/Delay'],'Value',num2str(Delay));
      | end
      mask Display: text(0.5,0.5,['z^{ ' num2str((-1)*str2double(get_param(gcb,'Delay'))) '}'],'texmode','on');
  Rp delay : Subsystem  TreatAsAtomicUnit=on  mask{Delay=0}
      mask prompts: Delay "Delay (in simulation steps) for the input signal:"
      mask init:
      | %set_param([gcb '/Discrete Transfer Fcn'],'Denominator',['[' num2str([1 zeros(1,str2double(get_param(gcb,'Delay')))]) ']']);
      mask CallbackString:
      | Delay = str2double(get_param(gcb,'Delay'));
      | if Delay < 0
      |     set_param(gcb,'Delay','0');
      |     error('Only non-negative delays are possible (causality).');
      |     set_param([gcb '/Delay'],'Value','0');
      | elseif Delay == 0
      |     set_param([gcb '/Delay'],'Value','0');
      | else
      |     set_param([gcb '/Integer Delay'],'NumDelays',num2str(Delay));
      |     set_param([gcb '/Delay'],'Value',num2str(Delay));
      | end
      mask Display: text(0.5,0.5,['z^{ ' num2str((-1)*str2double(get_param(gcb,'Delay'))) '}'],'texmode','on');
  Ta delay : Subsystem  TreatAsAtomicUnit=on  mask{Delay=0}
      mask prompts: Delay "Delay (in simulation steps) for the input signal:"
      mask init:
      | %set_param([gcb '/Discrete Transfer Fcn'],'Denominator',['[' num2str([1 zeros(1,str2double(get_param(gcb,'Delay')))]) ']']);
      mask CallbackString:
      | Delay = str2double(get_param(gcb,'Delay'));
      | if Delay < 0
      |     set_param(gcb,'Delay','0');
      |     error('Only non-negative delays are possible (causality).');
      |     set_param([gcb '/Delay'],'Value','0');
      | elseif Delay == 0
      |     set_param([gcb '/Delay'],'Value','0');
      | else
      |     set_param([gcb '/Integer Delay'],'NumDelays',num2str(Delay));
      |     set_param([gcb '/Delay'],'Value',num2str(Delay));
      | end
      mask Display: text(0.5,0.5,['z^{ ' num2str((-1)*str2double(get_param(gcb,'Delay'))) '}'],'texmode','on');
  Tp delay : Subsystem  TreatAsAtomicUnit=on  mask{Delay=0}
      mask prompts: Delay "Delay (in simulation steps) for the input signal:"
      mask init:
      | %set_param([gcb '/Discrete Transfer Fcn'],'Denominator',['[' num2str([1 zeros(1,str2double(get_param(gcb,'Delay')))]) ']']);
      mask CallbackString:
      | Delay = str2double(get_param(gcb,'Delay'));
      | if Delay < 0
      |     set_param(gcb,'Delay','0');
      |     error('Only non-negative delays are possible (causality).');
      |     set_param([gcb '/Delay'],'Value','0');
      | elseif Delay == 0
      |     set_param([gcb '/Delay'],'Value','0');
      | else
      |     set_param([gcb '/Integer Delay'],'NumDelays',num2str(Delay));
      |     set_param([gcb '/Delay'],'Value',num2str(Delay));
      | end
      mask Display: text(0.5,0.5,['z^{ ' num2str((-1)*str2double(get_param(gcb,'Delay'))) '}'],'texmode','on');
  V delay : Subsystem  TreatAsAtomicUnit=on  mask{Delay=0}
      mask prompts: Delay "Delay (in simulation steps) for the input signal:"
      mask init:
      | %set_param([gcb '/Discrete Transfer Fcn'],'Denominator',['[' num2str([1 zeros(1,str2double(get_param(gcb,'Delay')))]) ']']);
      mask CallbackString:
      | Delay = str2double(get_param(gcb,'Delay'));
      | if Delay < 0
      |     set_param(gcb,'Delay','0');
      |     error('Only non-negative delays are possible (causality).');
      |     set_param([gcb '/Delay'],'Value','0');
      | elseif Delay == 0
      |     set_param([gcb '/Delay'],'Value','0');
      | else
      |     set_param([gcb '/Integer Delay'],'NumDelays',num2str(Delay));
      |     set_param([gcb '/Delay'],'Value',num2str(Delay));
      | end
      mask Display: text(0.5,0.5,['z^{ ' num2str((-1)*str2double(get_param(gcb,'Delay'))) '}'],'texmode','on');
  error : Subsystem
  none - pass - fail : Subsystem
  sw D : Switch  Criteria=u2 ~= 0
  sw V : Switch  Criteria=u2 ~= 0
  VF Info : Outport  OutDataType=sfix(16)  OutScaling=2^0
  wires:
  V/1 -> Bus Selector/1, Bus Selector1/1, Bus Assignment1/1
  error/1(Verror) -> sw V/2, sw D/2
  Constant/1 -> sw V/1
  none - pass - fail/1(Verdict) -> sw V/3
  none - pass - fail/2(MaxDelay) -> sw D/1
  none - pass - fail/3(Delay) -> sw D/3
  sw V/1 -> Bus Assignment/2
  sw D/1 -> Bus Assignment/3
  Bus Selector/1 -> V delay/1(In1), Ra delay/1(In1), Ta delay/1(In1)  "<Local verdict>"
  Bus Assignment/1 -> VF Info/1
  Bus Selector2/1 -> Rp delay/1(In1)  "<R>"
  Bus Selector2/2 -> Tp delay/1(In1)  "<T>"
  Bus Selector2/3 -> A delay/1(In1)  "<A>"
  Rp delay/1(Out1) -> error/1(Rp), none - pass - fail/1(Rp), AND1/1
  Tp delay/1(Out1) -> error/2(Tp), none - pass - fail/2(Tp)
  A delay/1(Out1) -> error/3(A), none - pass - fail/3(A)
  V delay/1(Out1) -> error/6(V), none - pass - fail/6(V)
  Ra delay/1(Out1) -> none - pass - fail/4(Ra), AND1/2, error/4(Ra)
  AND1/1 -> none - pass - fail/7(R AND)
  Precond/1 -> Bus Selector2/1
  Bus Selector1/1 -> Delay bus signals/1(ELLin)  "<Expected lower limit>"
  Bus Selector1/2 -> Delay bus signals/2(EULin)  "<Expected upper limit>"
  Bus Selector1/3 -> Delay bus signals/3(ADin)  "<Actual data>"
  Bus Assignment1/1 -> Bus Assignment/1
  Delay bus signals/1(ELLout) -> Bus Assignment1/2
  Delay bus signals/2(EULout) -> Bus Assignment1/3
  Delay bus signals/3(ADout) -> Bus Assignment1/4
  Ta delay/1(Out1) -> none - pass - fail/5(Ta), error/5(Ta)

== system Pedal_Interpretation_exe/Validation Functions/SR-PI-01.1 Brake Pedal recognition/BrakePedal == 1/Range - Gap Relative tolerance Ass ==
  Signal : Inport  OutDataType=sfix(16)  OutScaling=2^0
  Reference : Inport  Port=2  OutDataType=sfix(16)  OutScaling=2^0
  Abs : Abs
  Abs1 : Abs
  Add : Sum  Inputs=+-  OutDataType=sfix(16)  OutScaling=2^-10
  Add1 : Sum  Inputs=+-  OutDataType=sfix(16)  OutScaling=2^-10
  Add2 : Sum  OutDataType=sfix(16)  OutScaling=2^-10
  Bus Creator : BusCreator  Inputs=5
  Data Type Conversion : DataTypeConversion  OutDataTypeMode=double  OutDataType=sfix(16)  OutScaling=2^0
  Data Type Conversion1 : DataTypeConversion  OutDataType=sfix(16)  OutScaling=2^0
  Data Type Conversion2 : DataTypeConversion  OutDataType=sfix(16)  OutScaling=2^0
  Data Type Conversion3 : DataTypeConversion  OutDataType=sfix(16)  OutScaling=2^0
  Delay : Constant  Value=0  OutDataType=sfix(16)  OutScaling=2^0
  Divide1 : Product  Inputs=**/  OutDataType=sfix(16)  OutScaling=2^-10
  Max : Constant  Value=100  OutDataType=sfix(16)  OutScaling=2^0
  Relational Operator : RelationalOperator  Operator=<=  LogicOutDataTypeMode=boolean
  Relative Tolerance : Constant  OutDataType=sfix(16)  OutScaling=2^0
  V : Outport  OutDataType=sfix(16)  OutScaling=2^0  InitialOutput=[2]
  wires:
  Data Type Conversion3/1 -> Bus Creator/4  "Actual data"
  Data Type Conversion2/1 -> Bus Creator/3  "Expected upper limit"
  Data Type Conversion1/1 -> Bus Creator/2  "Expected lower limit"
  Data Type Conversion/1 -> Bus Creator/1  "Local verdict"
  Bus Creator/1 -> V/1
  Add1/1 -> Data Type Conversion1/1
  Add2/1 -> Data Type Conversion2/1
  Delay/1 -> Bus Creator/5  "Delay"
  Abs1/1 -> Divide1/1
  Relational Operator/1 -> Data Type Conversion/1
  Relative Tolerance/1 -> Divide1/2
  Max/1 -> Divide1/3
  Divide1/1 -> Add2/1, Add1/2, Relational Operator/2
  Reference/1 -> Add1/1, Add2/2, Abs1/1, Add/2
  Signal/1 -> Data Type Conversion3/1, Add/1
  Add/1 -> Abs/1
  Abs/1 -> Relational Operator/1
